simulink model "generate_cartesian_velocity_motion"  (R2021a)
settings: Solver=FixedStepDiscrete  StartTime=0.0  StopTime=inf  FixedStep=0.001  RelTol=1e-3  EnableMultiTasking=on
PreLoadFcn:
  | set_param(gcs, 'RTWSystemTargetFile', 'franka_emika_panda.tlc');
  | demos_common_configs();
  | 
  | collision_behavior = ...
  |             [25.0, 25.0, 22.0, 20.0, 19.0, 17.0, 14.0,... % lower_torque_thresholds_acceleration
  |              35.0, 35.0, 32.0, 30.0, 29.0, 27.0, 24.0,... % upper_torque_thresholds_acceleration
  |              25.0, 25.0, 22.0, 20.0, 19.0, 17.0, 14.0,... % lower_torque_thresholds_nominal
  |              35.0, 35.0, 32.0, 30.0, 29.0, 27.0, 24.0,... % upper_torque_thresholds_nominal
  |              30.0, 30.0, 30.0, 25.0, 25.0, 25.0,...       % lower_force_thresholds_acceleration
  |              40.0, 40.0, 40.0, 35.0, 35.0, 35.0,...       % upper_force_thresholds_acceleration
  |              30.0, 30.0, 30.0, 25.0, 25.0, 25.0,...       % lower_force_thresholds_nominal
  |              40.0, 40.0, 40.0, 35.0, 35.0, 35.0];         % upper_force_thresholds_nominal
values from neighbouring files (symbols this model uses):
  amp = 0.5    [demos_common_configs.m]
  dof = 5    [demos_common_configs.m]
  init_delay = 10    [demos_common_configs.m]
  tuning_signal = 4    [demos_common_configs.m]
libraries: simulink x3, franka_simulink_library x2
settings Model: SimulationMode=external  ExtModeTrigDuration=10000  Creator=vasi_ko  LastModifiedBy=host
settings SolverCC: AlgebraicLoopSolver=TrustRegion
settings DataIOCC: LimitDataPoints=on  SaveFormat=Array  ReturnWorkspaceOutputs=off
settings OptimizationCC: DefaultParameterBehavior=Inlined  EnhancedBackFolding=on  PassReuseOutputArgsThreshold=0  OptimizeBlockOrder=speed  DifferentSizesBufferReuse=on  OptimizationCustomize=off
settings DebuggingCC: SolverPrmCheckMsg=warning  ParameterTunabilityLossMsg=error  SFUnexpectedBacktrackingDiag=warning  SFNoUnconditionalDefaultTransitionDiag=warning  SFExecutionAtInitializationDiag=none  SFMachineParentedDataDiag=warning  ArithmeticOperatorsInVariantConditions=warning
settings HardwareCC: ProdBitPerLong=64  ProdHWDeviceType=Intel->x86-64 (Linux 64)
settings ModelReferenceCC: PropagateSignalLabelsOutOfModel=off
settings SFSimCC: SimUseLocalCustomCode=off  MATLABDynamicMemAlloc=off  CustomCodeUndefinedFunction=UseInterfaceOnly  SimTargetLang=C++
settings RTWCC: Description=Generic Real-Time Target  SystemTargetFile=franka_emika_panda.tlc  RTWVerbose=off  RTWUseLocalCustomCode=off  Toolchain=Franka Simulink | gmake (64-bit linux)  BuildConfiguration=Faster Runs  TargetLang=C++
settings CodeAppCC: ForceParamTrailComments=on  OperatorAnnotations=on
settings STFCustomTargetCC: TargetLangStandard=C99 (ISO)  ModelReferenceCompliant=off  MatFileLogging=on  SystemTargetFile=franka_emika_panda.tlc
settings GRTTargetCC: ModelReferenceCompliant=off  ParMdlRefBuildCompliant=off  CompOptLevelCompliant=off  ConcurrentExecutionCompliant=off  CombineOutputUpdateFcns=off  CPPClassGenCompliant=off  GRTInterface=on  ExtModeStaticAlloc=on  ExtModeTransport=1  ExtModeMexFile=ext_xcp  ExtModeIntrfLevel=Level2 - Open
settings ConfigComp: CovMetricSettings=dw  CovSaveCumulativeToWorkspaceVar=on  CovSaveSingleToWorkspaceVar=on  CovExternalEMLEnable=off  CovSFcnEnable=off

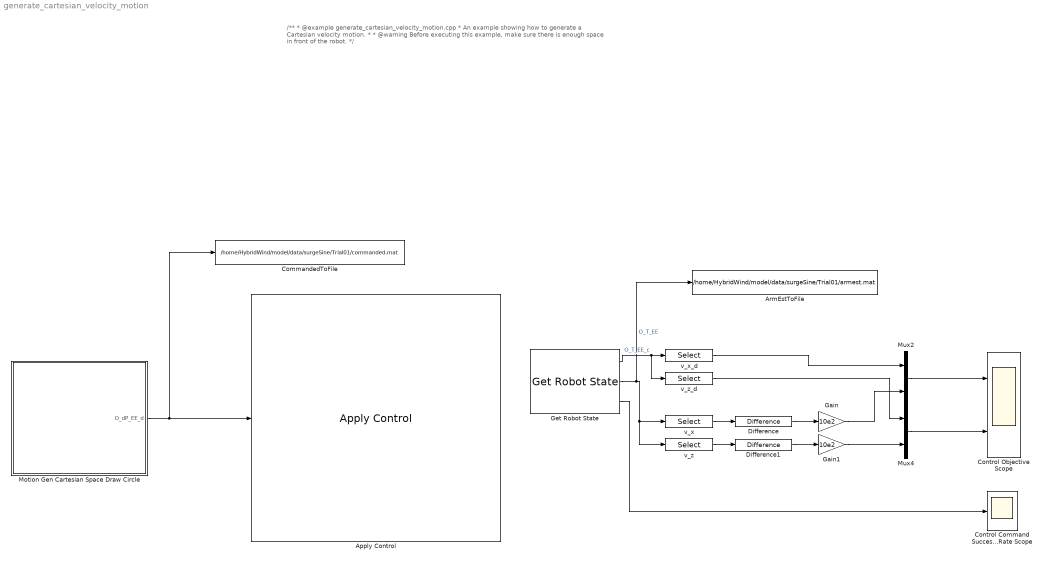
== system generate_cartesian_velocity_motion ==
  note: /**
      |  * @example generate_cartesian_velocity_motion.cpp
      |  * An example showing how to generate a Cartesian velocity motion.
      |  *
      |  * @warning Before executing this example, make sure there is enough space in front of the robot.
      |  */
  Apply Control : franka_simulink_library/Apply Control  robot_ip=robot_ip  gripper_attached=off  control_mode=Cartesian Velocities - Internal Controller Mode  controller_choice=Joint Impedance Controller  elbow_control=off  collision_thresholds=[25.0, 25.0, 22.0, 20.0, 19.0, 17.0, 14.0,35.0, 35.0, 32.0, 30.0, 29.0, 27.0, 24.0,25.0, 25.0, 22.0, 20.0, 19.0, 17.0, 14.0,35.0, 35.0, 32.0, 30.0, 29.0, 27.0, 24.0,30.0, 30.0, 30.0, 25.0, 25.0, 25.0,40.0, 40.0, 40.0, 35.0, 35.0, 35.0,30.0, 30.0, 30.0, 25.0, 25.0, 25.0,40.0, 40.0, 40.0, 35.0, 35.0, 35.0]  joint_impedance=[3000, 3000, 3000, 2500, 2500, 2000, 2000]  cartesian_impedance=cartesian_impedance  load_inertia=load_inertia  EE_T_K=EE_T_K  init_joint_configuration_req=on  init_joint_configuration=q_init
      settings: SourceProductName=Franka Emika
  ArmEstToFile : ToFile  Filename=/home/HybridWind/model/data/surgeSine/Trial01/armest.mat  MatrixName=armest
  CommandedToFile : ToFile  Filename=/home/HybridWind/model/data/surgeSine/Trial01/commanded.mat  MatrixName=commanded
  Control Command Success Rate Scope : Scope
  Control Objective Scope : Scope  NumInputPorts=2
  Difference : simulink/Discrete/Difference  ICPrevInput=0.3069  OutMin=[]  OutMax=[]  OutDataType=fixdt(1, 16)  OutScaling=2^-10  DoSatur=off
  Difference1 : simulink/Discrete/Difference  ICPrevInput=0.5902  OutMin=[]  OutMax=[]  OutDataType=fixdt(1, 16)  OutScaling=2^-10  DoSatur=off
  Gain : Gain  Gain=10e2
  Gain1 : Gain  Gain=10e2
  Get Robot State : franka_simulink_library/Get Robot State  robot_ip=robot_ip  signals_requested='O_dP_EE_c O_T_EE control_command_success_rate'
      settings: SourceProductName=Franka Emika
  Motion Gen Cartesian Space Draw Circle : Subsystem
      mask Display:
      | pos = get_param(gcb, 'Position');
      | width = pos(3) - pos(1);
      | x = [0:width];
      | y = sin(x/180*pi);
      | % Parameters 'm' and 'b' must be defined in 'Parameters & Dialog' pane.
      | plot((1/2)*cos(x/180*2*pi+pi/4), (1/2)*sin(x/180*2*pi+pi/4));
      | 
      | port_label('output',1,'O_dP_EE_d');
  Mux2 : Mux  Inputs=2
  Mux4 : Mux  Inputs=2
  v_x : Selector  InputPortWidth=16  IndexOptions=Index vector (dialog)  Indices=13  OutputSizes=1
  v_x_d : Selector  InputPortWidth=6  IndexOptions=Index vector (dialog)  Indices=1  OutputSizes=1
  v_z : Selector  InputPortWidth=16  IndexOptions=Index vector (dialog)  Indices=15  OutputSizes=1
  v_z_d : Selector  InputPortWidth=6  IndexOptions=Index vector (dialog)  Indices=3  OutputSizes=1
  wires:
  Motion Gen Cartesian Space Draw Circle/1(O_dP_EE_d) -> CommandedToFile/1, Apply Control/1
  Get Robot State/1 -> v_x_d/1, v_z_d/1  "O_T_EE_c"
  Get Robot State/2 -> ArmEstToFile/1, v_z/1, v_x/1  "O_T_EE"
  v_x/1 -> Difference/1
  v_z/1 -> Difference1/1
  Difference/1 -> Gain/1
  Difference1/1 -> Gain1/1
  Gain1/1 -> Mux4/2
  Gain/1 -> Mux2/2
  v_x_d/1 -> Mux2/1
  v_z_d/1 -> Mux4/1
  Mux2/1 -> Control Objective Scope/1
  Mux4/1 -> Control Objective Scope/2
  Get Robot State/3 -> Control Command Success Rate Scope/1

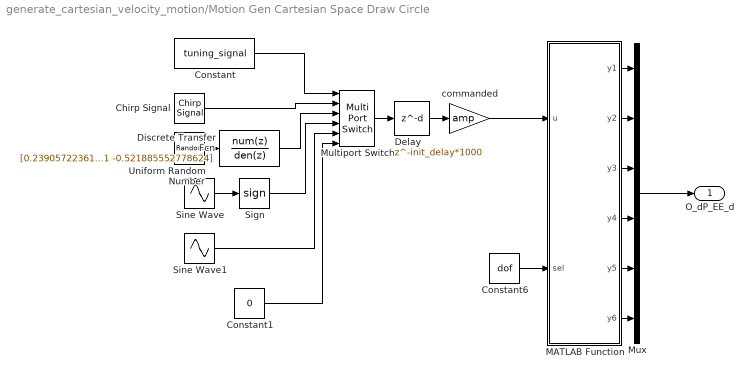
== system generate_cartesian_velocity_motion/Motion Gen Cartesian Space Draw Circle ==
  Chirp Signal : simulink/Sources/Chirp Signal  f1=0.1  T=60  f2=20
  Constant : Constant  Value=tuning_signal
  Constant1 : Constant  Value=0
  Constant6 : Constant  Value=dof
  Delay : Delay  DelayLength=init_delay*1000
  Discrete Transfer Fcn : DiscreteTransferFcn  Numerator=[0.239057223610688 0.239057223610688]  Denominator=[1 -0.521885552778624]
  MATLAB Function : MATLAB Function  TreatAsAtomicUnit=on
  Multiport Switch : MultiPortSwitch  Inputs=5
  Mux : Mux  Inputs=6
  Sign : Signum
  Sine Wave : Sin  Amplitude=amp  Frequency=2*pi/60  SampleTime=0
  Sine Wave1 : Sin  Amplitude=amp  Frequency=2*pi/1  SampleTime=0
  Uniform Random Number : UniformRandomNumber  SampleTime=0.001
  commanded : Gain  Gain=amp
  O_dP_EE_d : Outport  VectorParamsAs1DForOutWhenUnconnected=off
  wires:
  Uniform Random Number/1 -> Discrete Transfer Fcn/1
  MATLAB Function/6(y6) -> Mux/6
  MATLAB Function/5(y5) -> Mux/5
  commanded/1 -> MATLAB Function/1(u)
  MATLAB Function/3(y3) -> Mux/3
  MATLAB Function/2(y2) -> Mux/2
  Sign/1 -> Multiport Switch/4
  Sine Wave/1 -> Sign/1
  Delay/1 -> commanded/1
  MATLAB Function/4(y4) -> Mux/4
  Constant6/1 -> MATLAB Function/2(sel)
  Multiport Switch/1 -> Delay/1
  Discrete Transfer Fcn/1 -> Multiport Switch/3
  MATLAB Function/1(y1) -> Mux/1
  Constant/1 -> Multiport Switch/1
  Constant1/1 -> Multiport Switch/6
  Chirp Signal/1 -> Multiport Switch/2
  Mux/1 -> O_dP_EE_d/1
  Sine Wave1/1 -> Multiport Switch/5

== matlab function generate_cartesian_velocity_motion/Motion Gen Cartesian Space Draw Circle/MATLAB Function ==
  data: u input; y1 output; sel input; y2 output; y3 output; y4 output; y5 output; y6 output
function [y1, y2, y3, y4, y5, y6] = fcn(u, sel)

y1 = 0;
y2 = 0;
y3 = 0;
y4 = 0;
y5 = 0;
y6 = 0;

switch sel
    case 1
        y1 = u;
    case 2
        y2 = u;
    case 3
        y3 = u;
    case 4
        y4 = u;
    case 5
        y5 = u;
    case 6
        y6 = u;
    otherwise
        y1 = 0;
end
